simulink model "untitled"  (R2024b)
settings: Solver=VariableStepAuto  StartTime=0.0  StopTime=10.0  RelTol=1e-3
libraries: simulink x1
settings Model: Creator=10537  LastModifiedBy=10537

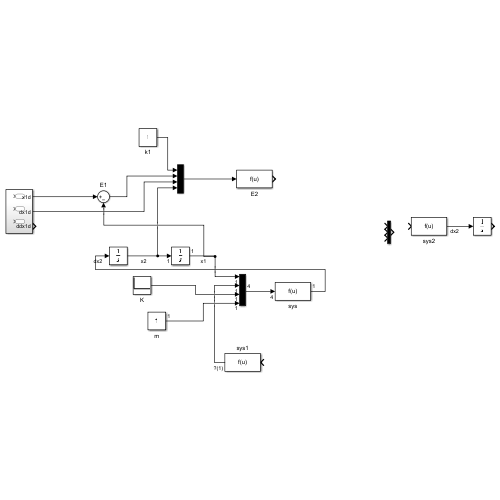
[thumbnail: Simulink's stored preview of the top-level diagram]
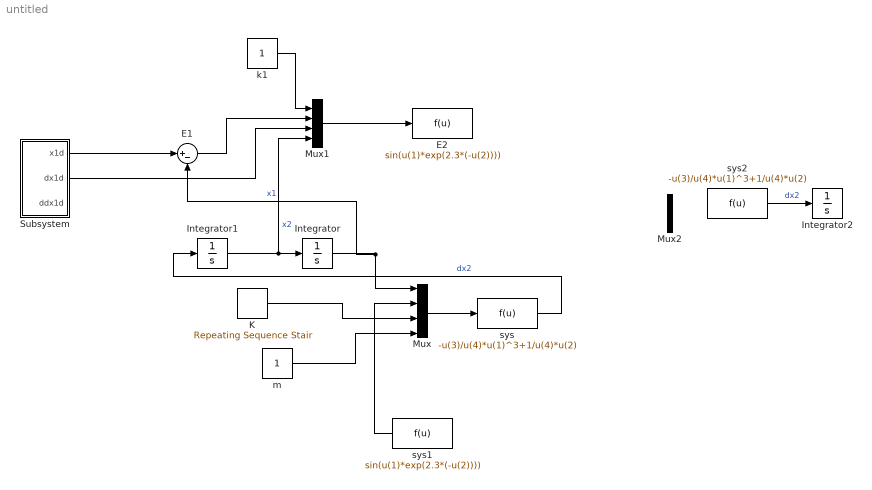
== system untitled ==
  E1 : Sum  Inputs=|+-
  E2 : Fcn  Expr=sin(u(1)*exp(2.3*(-u(2))))
  Integrator : Integrator
  Integrator1 : Integrator
  Integrator2 : Integrator
  K : simulink/Sources/Repeating Sequence Stair  OutValues=8  tsamp=20  OutMin=[]  OutMax=[]  OutDataTypeStr=double  OutputDataTypeScalingMode=double  OutDataType=fixdt(0,8)  ConRadixGroup=Best Precision: Vector-wise  OutScaling=2^-12
  Mux : Mux
  Mux1 : Mux
  Mux2 : Mux  Inputs=3
  Subsystem : Subsystem
  k1 : Constant
  m : Constant
  sys : Fcn  Expr=-u(3)/u(4)*u(1)^3+1/u(4)*u(2)
  sys1 : Fcn  Expr=sin(u(1)*exp(2.3*(-u(2))))
  sys2 : Fcn  Expr=-u(3)/u(4)*u(1)^3+1/u(4)*u(2)
  wires:
  Integrator/1 -> E1/2, Mux/1  "x1"
  Mux/1 -> sys/1
  m/1 -> Mux/4
  K/1 -> Mux/3
  Integrator1/1 -> Mux1/4, Integrator/1  "x2"
  sys/1 -> Integrator1/1  "dx2"
  Subsystem/1(x1d) -> E1/1
  sys1/1 -> Mux/2
  Subsystem/2(dx1d) -> Mux1/3
  k1/1 -> Mux1/1
  E1/1 -> Mux1/2
  Mux1/1 -> E2/1
  sys2/1 -> Integrator2/1  "dx2"

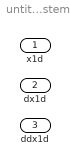
== system untitled/Subsystem ==
  x1d : Outport
  dx1d : Outport  Port=2
  ddx1d : Outport  Port=3
